simulink model "Vehicle_Model_noLT"  (R2020a)
settings: Solver=VariableStepAuto  StartTime=0.0  StopTime=inf  RelTol=1e-3
PreLoadFcn:
  | data_struct=load('Torque_curve.mat');
  | data=data_struct.torque;
  | breakpoints1=data(:,1);
  | table_data=data(:,2);
InitFcn:
  | Coeff_long_C=load('Tire model/pacejka_coefficients_longitudinal.mat');
  | Coeff_long=Coeff_long_C.C;
  | Coeff_lat_C=load('Tire model/pacejka_coefficients_lateral.mat');
  | Coeff_lat=Coeff_lat_C.C;
values from neighbouring files (symbols this model uses):
  Car_Iz = 145.0    [Properties.sldd]
  Car_mass = 245.0    [Properties.sldd]
  CG_x = 0.6    [Properties.sldd]
  Initial_speed = 15.0    [Properties.sldd]
  Track_width = 2.0    [Properties.sldd]
  Wheelbase = 1.2    [Properties.sldd]
libraries: vehdynlibsteering x1
settings Model: DataDictionary=Properties.sldd  Creator=Matthew  LastModifiedBy=Matthew
settings DebuggingCC: ModelReferenceExtraNoncontSigs=warning
settings ModelReferenceCC: ModelReferenceMinAlgLoopOccurrences=on

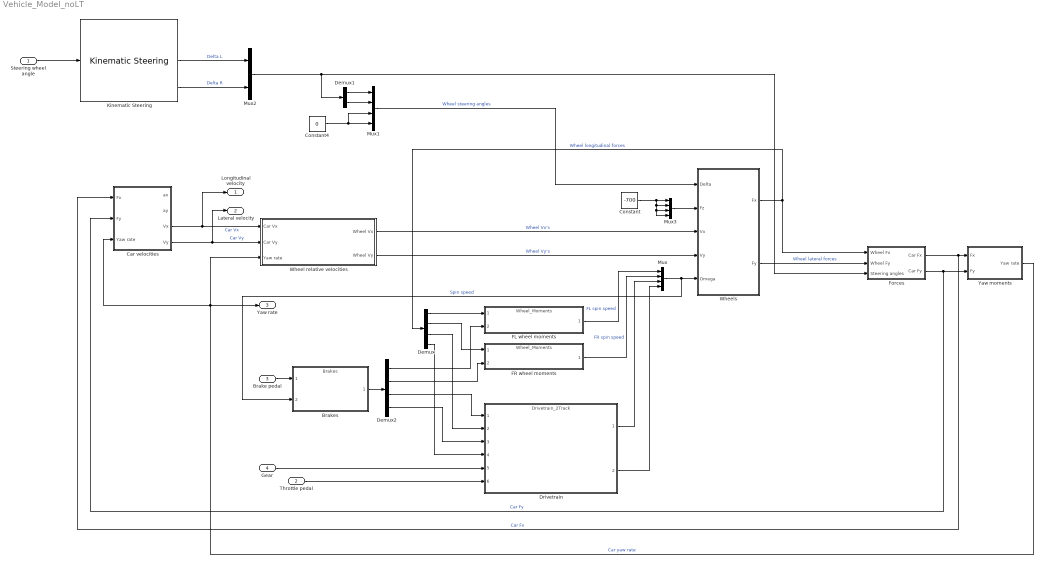
== system Vehicle_Model_noLT ==
  Steering wheel angle : Inport
  Throttle pedal : Inport  Port=2
  Brake pedal : Inport  Port=3
  Gear : Inport  Port=4
  Brakes : ModelReference  ModelNameDialog=Brakes  SimulationMode=Normal  ModelReferenceVersion=1.8
  Car velocities : Subsystem
  Constant : Constant  Value=-700
  Constant4 : Constant  Value=0
  Demux : Demux
  Demux1 : Demux  Outputs=2
  Demux2 : Demux
  Drivetrain : ModelReference  ModelNameDialog=Drivetrain_2Track.slx  SimulationMode=Normal  ModelReferenceVersion=1.31
  FL wheel moments : ModelReference  ModelNameDialog=Wheel_Moments  SimulationMode=Normal  ModelReferenceVersion=1.4
  FR wheel moments : ModelReference  ModelNameDialog=Wheel_Moments  SimulationMode=Normal  ModelReferenceVersion=1.4
  Forces : Subsystem
  Kinematic Steering : vehdynlibsteering/Kinematic Steering  StrgType=Rack and pinion  StrgRatioType=Constant  Loc=Front  NrmlFctr=0.01  TrckWdth=1  WhlBase=1.524  Db=0  StrgRng=1.25*pi  StrgAngBpts="[-6.2832   -5.0265   -3.7699   -2.5133   -1.2566         0    1.2566    2.5133    3.7699    5.0265    6.2832]"  StrgRatioTbl=|  StrgRatio=100  StrgArmLngth=0.1  RckCsLngth=0.5  TieRodLngth=0.248  D=0.2  PnnRadius=0.0057  PnnRadiusTbl="[0.0055    0.0055    0.0056    0.0057    0.0058    0.0057    0.0057    0.0057    0.0056    0.0055    0.0055]"  RodLngth=0.1  ParaArmLngth=0.9  aMode=2
      | [13.5000   13.3750   13.2500   13.1250   13.0000   13.0000   13.0000   13.1250   13.2500   13.3750   13.5000
      | ]
  Mux : Mux
  Mux1 : Mux
  Mux2 : Mux  Inputs=2
  Mux3 : Mux
  Wheel relative velocities : Subsystem
  Wheels : Subsystem
  Yaw moments : Subsystem
  Longitudinal velocity : Outport
  Lateral velocity : Outport  Port=2
  Yaw rate : Outport  Port=3
  wires:
  Mux/1 -> Brakes/2, Wheels/5(Omega)  "Spin speed"
  FL wheel moments/1 -> Mux/1  "FL spin speed"
  Demux1/1 -> Mux1/1
  Wheels/2(Fy) -> Forces/2(Wheel Fy)  "Wheel lateral forces"
  Drivetrain/2 -> Mux/4
  FR wheel moments/1 -> Mux/2  "FR spin speed"
  Demux1/2 -> Mux1/2
  Demux/3 -> Drivetrain/2
  Demux/1 -> FL wheel moments/1
  Wheel relative velocities/2(Wheel Vy) -> Wheels/4(Vy)  "Wheel Vy's"
  Drivetrain/1 -> Mux/3
  Gear/1 -> Drivetrain/5
  Wheels/1(Fx) -> Forces/1(Wheel Fx), Demux/1  "Wheel longitudinal forces"
  Forces/2(Car Fy) -> Yaw moments/2(Fy), Car velocities/2(Fy)  "Car Fy"
  Wheel relative velocities/1(Wheel Vx) -> Wheels/3(Vx)  "Wheel Vx's"
  Brake pedal/1 -> Brakes/1
  Demux/2 -> FR wheel moments/1
  Kinematic Steering/2 -> Mux2/1  "Delta L"
  Demux/4 -> Drivetrain/4
  Constant4/1 -> Mux1/4, Mux1/3
  Kinematic Steering/3 -> Mux2/2  "Delta R"
  Forces/1(Car Fx) -> Car velocities/1(Fx), Yaw moments/1(Fx)  "Car Fx"
  Yaw moments/1(Yaw rate) -> Wheel relative velocities/3(Yaw rate), Car velocities/3(Yaw rate), Yaw rate/1  "Car yaw rate"
  Mux2/1 -> Forces/3(Steering angles), Demux1/1
  Mux1/1 -> Wheels/1(Delta)  "Wheel steering angles"
  Car velocities/3(Vx) -> Longitudinal velocity/1, Wheel relative velocities/1(Car Vx)  "Car Vx"
  Car velocities/4(Vy) -> Lateral velocity/1, Wheel relative velocities/2(Car Vy)  "Car Vy"
  Throttle pedal/1 -> Drivetrain/6
  Mux3/1 -> Wheels/2(Fz)
  Constant/1 -> Mux3/2, Mux3/3, Mux3/4, Mux3/1
  Steering wheel angle/1 -> Kinematic Steering/1
  Demux2/1 -> FL wheel moments/2
  Demux2/2 -> FR wheel moments/2
  Demux2/3 -> Drivetrain/1
  Demux2/4 -> Drivetrain/3
  Brakes/1 -> Demux2/1

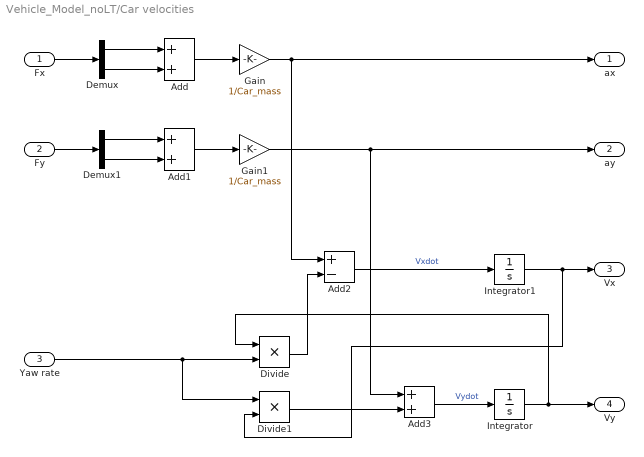
== system Vehicle_Model_noLT/Car velocities ==
  Fx : Inport
  Fy : Inport  Port=2
  Yaw rate : Inport  Port=3
  Add : Sum  Inputs=2
  Add1 : Sum  Inputs=2
  Add2 : Sum  Inputs=+-
  Add3 : Sum
  Demux : Demux  Outputs=2
  Demux1 : Demux  Outputs=2
  Divide : Product  Inputs=**
  Divide1 : Product  Inputs=**
  Gain : Gain  Gain=1/Car_mass
  Gain1 : Gain  Gain=1/Car_mass
  Integrator : Integrator
  Integrator1 : Integrator  InitialCondition=Initial_speed
  ax : Outport
  ay : Outport  Port=2
  Vx : Outport  Port=3
  Vy : Outport  Port=4
  wires:
  Fx/1 -> Demux/1
  Demux/1 -> Add/1
  Demux/2 -> Add/2
  Fy/1 -> Demux1/1
  Demux1/1 -> Add1/1
  Demux1/2 -> Add1/2
  Add/1 -> Gain/1
  Add1/1 -> Gain1/1
  Gain/1 -> ax/1, Add2/1
  Gain1/1 -> Add3/1, ay/1
  Integrator1/1 -> Divide1/2, Vx/1
  Integrator/1 -> Vy/1, Divide/1
  Yaw rate/1 -> Divide1/1, Divide/2
  Divide/1 -> Add2/2
  Divide1/1 -> Add3/2
  Add3/1 -> Integrator/1  "Vydot"
  Add2/1 -> Integrator1/1  "Vxdot"

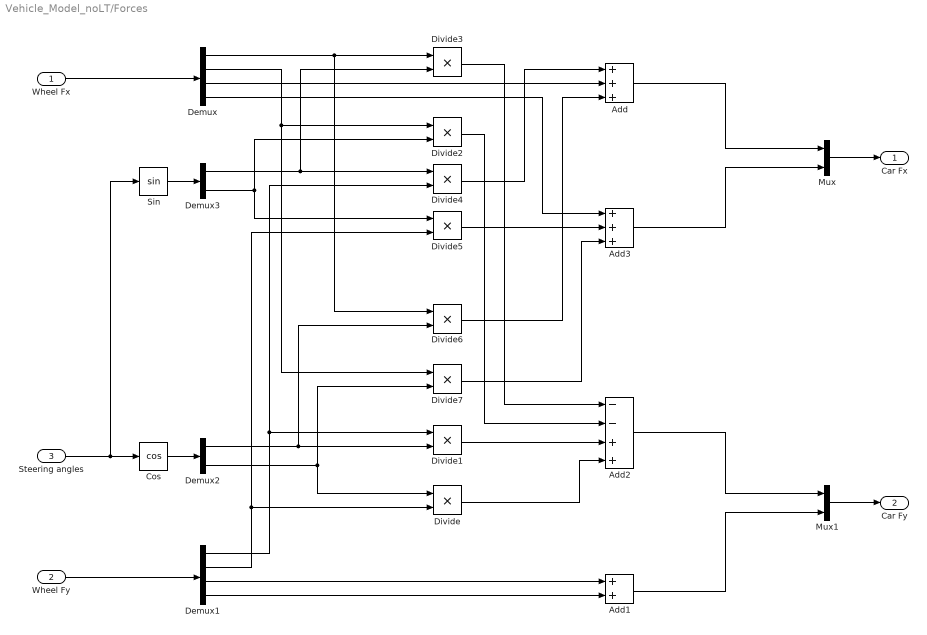
== system Vehicle_Model_noLT/Forces ==
  Wheel Fx : Inport
  Wheel Fy : Inport  Port=2
  Steering angles : Inport  Port=3
  Add : Sum  Inputs=3
  Add1 : Sum  Inputs=2
  Add2 : Sum  Inputs=--++
  Add3 : Sum  Inputs=3
  Cos : Trigonometry  Operator=cos
  Demux : Demux
  Demux1 : Demux
  Demux2 : Demux  Outputs=2
  Demux3 : Demux  Outputs=2
  Divide{,1..3,6..7} (6 alike) : Product  Inputs=**
  Divide4 : Product
  Divide5 : Product
  Mux : Mux  Inputs=2
  Mux1 : Mux  Inputs=2
  Sin : Trigonometry
  Car Fx : Outport
  Car Fy : Outport  Port=2
  wires:
  Wheel Fx/1 -> Demux/1
  Wheel Fy/1 -> Demux1/1
  Steering angles/1 -> Sin/1, Cos/1
  Cos/1 -> Demux2/1
  Demux2/2 -> Divide/1, Divide7/2
  Demux1/1 -> Divide1/1, Divide4/2
  Demux1/2 -> Divide5/2, Divide/2
  Demux2/1 -> Divide6/2, Divide1/2
  Sin/1 -> Demux3/1
  Demux3/1 -> Divide4/1, Divide3/2
  Demux/1 -> Divide6/1, Divide3/1
  Demux/2 -> Divide7/1, Divide2/1
  Demux3/2 -> Divide5/1, Divide2/2
  Demux/3 -> Add/2
  Demux1/3 -> Add1/1
  Demux1/4 -> Add1/2
  Add1/1 -> Mux1/2
  Add2/1 -> Mux1/1
  Add/1 -> Mux/1
  Add3/1 -> Mux/2
  Mux/1 -> Car Fx/1
  Mux1/1 -> Car Fy/1
  Demux/4 -> Add3/1
  Divide3/1 -> Add2/1
  Divide6/1 -> Add/3
  Divide5/1 -> Add3/2
  Divide4/1 -> Add/1
  Divide2/1 -> Add2/2
  Divide7/1 -> Add3/3
  Divide1/1 -> Add2/3
  Divide/1 -> Add2/4

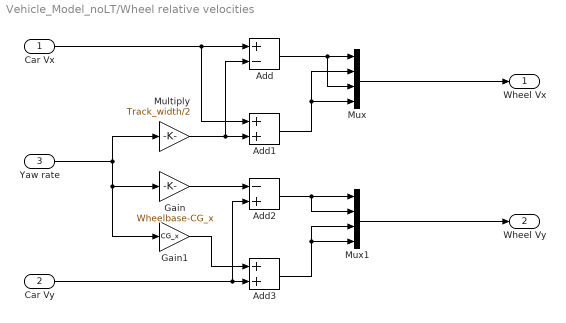
== system Vehicle_Model_noLT/Wheel relative velocities ==
  Car Vx : Inport
  Car Vy : Inport  Port=2
  Yaw rate : Inport  Port=3
  Add : Sum  Inputs=+-
  Add1 : Sum  Inputs=2
  Add2 : Sum  Inputs=-+
  Add3 : Sum  Inputs=2
  Gain : Gain  Gain=Wheelbase-CG_x
  Gain1 : Gain  Gain=CG_x
  Multiply : Gain  Gain=Track_width/2
  Mux : Mux
  Mux1 : Mux
  Wheel Vx : Outport
  Wheel Vy : Outport  Port=2
  wires:
  Yaw rate/1 -> Multiply/1, Gain1/1, Gain/1
  Car Vx/1 -> Add1/1, Add/1
  Multiply/1 -> Add1/2, Add/2
  Add/1 -> Mux/3, Mux/1
  Add1/1 -> Mux/4, Mux/2
  Mux/1 -> Wheel Vx/1
  Add3/1 -> Mux1/3, Mux1/4
  Gain/1 -> Add2/1
  Car Vy/1 -> Add2/2, Add3/2
  Add2/1 -> Mux1/2, Mux1/1
  Mux1/1 -> Wheel Vy/1
  Gain1/1 -> Add3/1

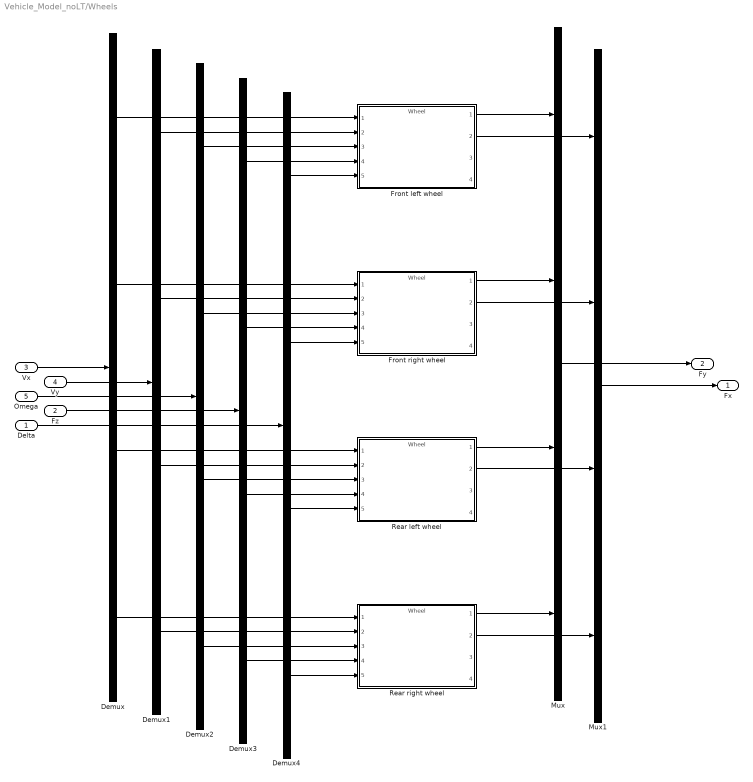
== system Vehicle_Model_noLT/Wheels ==
  Delta : Inport
  Fz : Inport  Port=2
  Vx : Inport  Port=3
  Vy : Inport  Port=4
  Omega : Inport  Port=5
  Demux{,1..4} (5 alike) : Demux
  Front left wheel : ModelReference  ModelNameDialog=Wheel  SimulationMode=Normal  ModelReferenceVersion=1.30
  Front right wheel : ModelReference  ModelNameDialog=Wheel  SimulationMode=Normal  ModelReferenceVersion=1.30
  Mux : Mux
  Mux1 : Mux
  Rear left wheel : ModelReference  ModelNameDialog=Wheel  SimulationMode=Normal  ModelReferenceVersion=1.30
  Rear right wheel : ModelReference  ModelNameDialog=Wheel  SimulationMode=Normal  ModelReferenceVersion=1.30
  Fx : Outport
  Fy : Outport  Port=2
  wires:
  Vx/1 -> Demux/1
  Fz/1 -> Demux3/1
  Delta/1 -> Demux4/1
  Vy/1 -> Demux1/1
  Omega/1 -> Demux2/1
  Demux/1 -> Front left wheel/1
  Demux1/1 -> Front left wheel/2
  Demux2/1 -> Front left wheel/3
  Demux3/1 -> Front left wheel/4
  Demux4/1 -> Front left wheel/5
  Demux4/2 -> Front right wheel/5
  Demux3/2 -> Front right wheel/4
  Demux2/2 -> Front right wheel/3
  Demux1/2 -> Front right wheel/2
  Demux/2 -> Front right wheel/1
  Demux/3 -> Rear left wheel/1
  Demux1/3 -> Rear left wheel/2
  Demux2/3 -> Rear left wheel/3
  Demux3/3 -> Rear left wheel/4
  Demux4/3 -> Rear left wheel/5
  Demux4/4 -> Rear right wheel/5
  Demux3/4 -> Rear right wheel/4
  Demux2/4 -> Rear right wheel/3
  Demux1/4 -> Rear right wheel/2
  Demux/4 -> Rear right wheel/1
  Front left wheel/1 -> Mux/1
  Front right wheel/1 -> Mux/2
  Rear left wheel/1 -> Mux/3
  Rear right wheel/1 -> Mux/4
  Mux/1 -> Fy/1
  Front left wheel/2 -> Mux1/1
  Front right wheel/2 -> Mux1/2
  Rear left wheel/2 -> Mux1/3
  Rear right wheel/2 -> Mux1/4
  Mux1/1 -> Fx/1

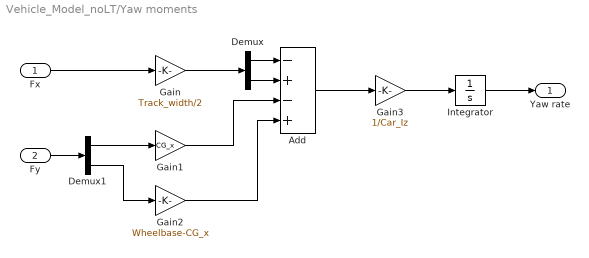
== system Vehicle_Model_noLT/Yaw moments ==
  Fx : Inport
  Fy : Inport  Port=2
  Add : Sum  Inputs=-+-+
  Demux : Demux  Outputs=2
  Demux1 : Demux  Outputs=2
  Gain : Gain  Gain=Track_width/2
  Gain1 : Gain  Gain=CG_x
  Gain2 : Gain  Gain=Wheelbase-CG_x
  Gain3 : Gain  Gain=1/Car_Iz
  Integrator : Integrator
  Yaw rate : Outport
  wires:
  Integrator/1 -> Yaw rate/1
  Fx/1 -> Gain/1
  Add/1 -> Gain3/1
  Gain/1 -> Demux/1
  Demux/1 -> Add/1
  Demux/2 -> Add/2
  Gain1/1 -> Add/3
  Fy/1 -> Demux1/1
  Demux1/1 -> Gain1/1
  Demux1/2 -> Gain2/1
  Gain2/1 -> Add/4
  Gain3/1 -> Integrator/1
